simulink model "model2_controller_observer"  (R2022b)
settings: Solver=VariableStepAuto  StartTime=0.0  StopTime=20  RelTol=1e-3
InitFcn:
  | model2_init_params_stable
values from neighbouring files (symbols this model uses):
  A_ccf = [ ... (first row only)    [model2_init_params_stable.m]    (also in model2_init_params_unstable.m; model2_init_params_unstable__lqr_controller.m)
  A_fobs = A_ccf-L*C_ccf    [model2_init_params_stable.m]    (also in model2_init_params_unstable.m)
  B_ccf = [ ... (first row only)    [model2_init_params_stable.m]    (also in model2_init_params_unstable.m; model2_init_params_unstable__lqr_controller.m)
  B_fobs = [B_ccf L]    [model2_init_params_stable.m]    (also in model2_init_params_unstable.m)
  C_ccf = [tf_num(5)  tf_num(4)   tf_num(3)   tf_num(2)]    [model2_init_params_stable.m]    (also in model2_init_params_unstable.m; model2_init_params_unstable__lqr_controller.m)
  C_fobs = eye(length(A_fobs))    [model2_init_params_stable.m]    (also in model2_init_params_unstable.m)
  D_ccf = 0    [model2_init_params_stable.m]    (also in model2_init_params_unstable.m; model2_init_params_unstable__lqr_controller.m)
  D_fobs = zeros(size(B_fobs))    [model2_init_params_stable.m]    (also in model2_init_params_unstable.m)
settings Model: Creator=neotod  LastModifiedBy=neotod

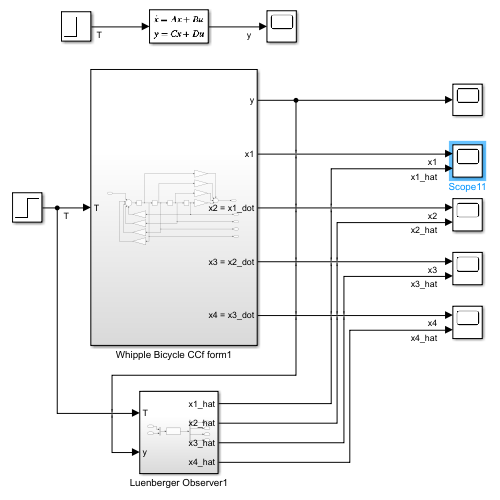
[thumbnail: Simulink's stored preview of the top-level diagram]
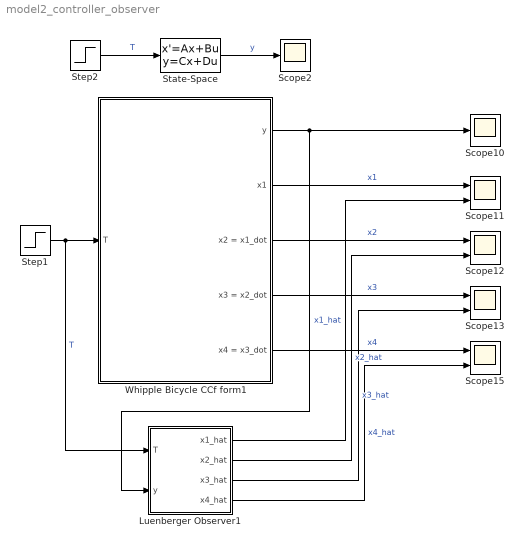
== system model2_controller_observer ==
  Luenberger Observer1 : Subsystem
  Scope10 : Scope
  Scope{11..13,15} (4 alike) : Scope  NumInputPorts=2
  Scope2 : Scope
  State-Space : StateSpace  A=A_ccf  B=B_ccf  C=C_ccf  D=D_ccf  InitialCondition=0
  Step1 : Step  Time=0.6  SampleTime=0
  Step2 : Step  SampleTime=0
  Whipple Bicycle CCf form1 : Subsystem
  wires:
  State-Space/1 -> Scope2/1  "y"
  Step2/1 -> State-Space/1  "T"
  Whipple Bicycle CCf form1/4(x3 = x2_dot) -> Scope13/1  "x3"
  Step1/1 -> Luenberger Observer1/1(T), Whipple Bicycle CCf form1/1(T)  "T"
  Whipple Bicycle CCf form1/5(x4 = x3_dot) -> Scope15/1  "x4"
  Whipple Bicycle CCf form1/2(x1) -> Scope11/1  "x1"
  Whipple Bicycle CCf form1/3(x2 = x1_dot) -> Scope12/1  "x2"
  Whipple Bicycle CCf form1/1(y) -> Luenberger Observer1/2(y), Scope10/1
  Luenberger Observer1/1(x1_hat) -> Scope11/2  "x1_hat"
  Luenberger Observer1/2(x2_hat) -> Scope12/2  "x2_hat"
  Luenberger Observer1/3(x3_hat) -> Scope13/2  "x3_hat"
  Luenberger Observer1/4(x4_hat) -> Scope15/2  "x4_hat"

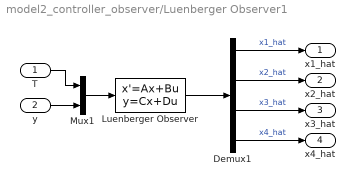
== system model2_controller_observer/Luenberger Observer1 ==
  T : Inport
  y : Inport  Port=2
  Demux1 : Demux
  Luenberger Observer : StateSpace  A=A_fobs  B=B_fobs  C=C_fobs  D=D_fobs  InitialCondition=0
  Mux1 : Mux  Inputs=2
  x1_hat : Outport
  x2_hat : Outport  Port=2
  x3_hat : Outport  Port=3
  x4_hat : Outport  Port=4
  wires:
  Demux1/2 -> x2_hat/1  "x2_hat"
  Mux1/1 -> Luenberger Observer/1
  Luenberger Observer/1 -> Demux1/1
  Demux1/1 -> x1_hat/1  "x1_hat"
  Demux1/3 -> x3_hat/1  "x3_hat"
  Demux1/4 -> x4_hat/1  "x4_hat"
  T/1 -> Mux1/1
  y/1 -> Mux1/2

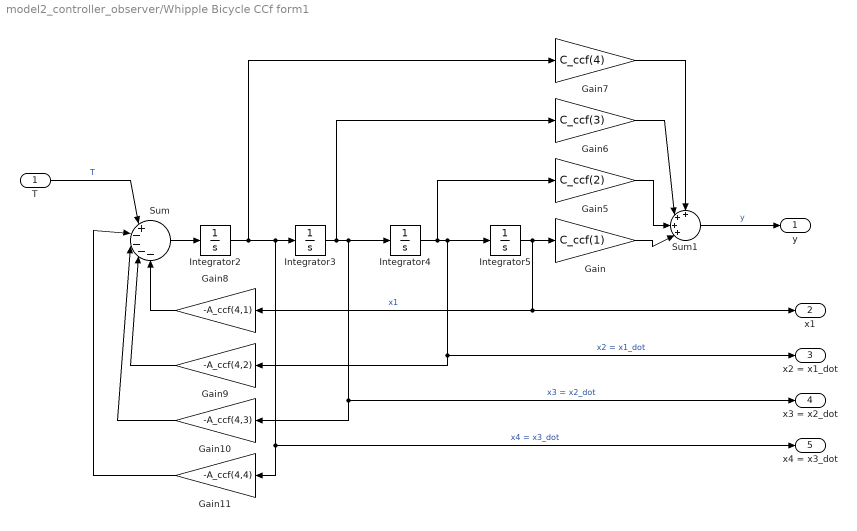
== system model2_controller_observer/Whipple Bicycle CCf form1 ==
  T : Inport
  Gain : Gain  Gain=C_ccf(1)
  Gain10 : Gain  Gain=-A_ccf(4,3)
  Gain11 : Gain  Gain=-A_ccf(4,4)
  Gain5 : Gain  Gain=C_ccf(2)
  Gain6 : Gain  Gain=C_ccf(3)
  Gain7 : Gain  Gain=C_ccf(4)
  Gain8 : Gain  Gain=-A_ccf(4,1)
  Gain9 : Gain  Gain=-A_ccf(4,2)
  Integrator{2..5} (4 alike) : Integrator
  Sum : Sum  Inputs=|+----
  Sum1 : Sum  Inputs=++++|
  y : Outport
  x1 : Outport  Port=2
  x2 = x1_dot : Outport  Port=3
  x3 = x2_dot : Outport  Port=4
  x4 = x3_dot : Outport  Port=5
  wires:
  Integrator3/1 -> Gain6/1, x3 = x2_dot/1, Gain10/1, Integrator4/1  "x3 = x2_dot"
  Gain7/1 -> Sum1/1
  Integrator2/1 -> Gain7/1, x4 = x3_dot/1, Gain11/1, Integrator3/1  "x4 = x3_dot"
  Integrator5/1 -> x1/1, Gain8/1, Gain/1  "x1"
  Gain10/1 -> Sum/3
  Integrator4/1 -> Gain5/1, x2 = x1_dot/1, Gain9/1, Integrator5/1  "x2 = x1_dot"
  Gain6/1 -> Sum1/2
  Sum1/1 -> y/1  "y"
  T/1 -> Sum/1  "T"
  Gain8/1 -> Sum/5
  Sum/1 -> Integrator2/1
  Gain5/1 -> Sum1/3
  Gain/1 -> Sum1/4
  Gain11/1 -> Sum/2
  Gain9/1 -> Sum/4
